simulink model "Espacio_Estados_sin_ROS_Comparacion"  (R2023a)
settings: Solver=VariableStepAuto  StartTime=0.0  StopTime=50  RelTol=1e-3
undefined symbols (not defined in the file): A, B, C, D, Ke, Ki
settings Model: Creator=mluser  LastModifiedBy=camarin
settings SolverCC: AlgebraicLoopSolver=TrustRegion
settings DataIOCC: ReturnWorkspaceOutputs=off
settings DebuggingCC: UnconnectedInputMsg=warning  UnconnectedOutputMsg=warning  UnconnectedLineMsg=warning
settings ModelReferenceCC: EnableRefExpFcnMdlSchedulingChecks=on
settings RTWCC: DLArmComputeVersion=19.05

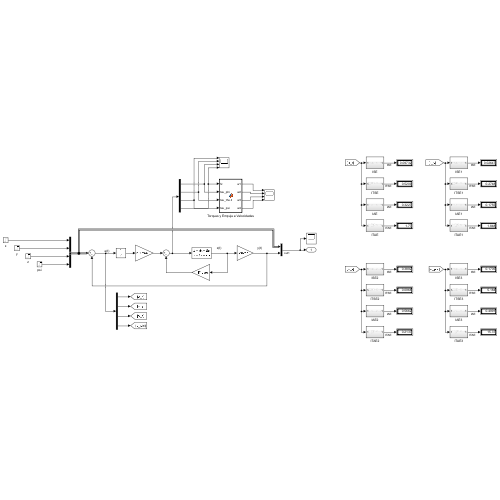
[thumbnail: Simulink's stored preview of the top-level diagram]
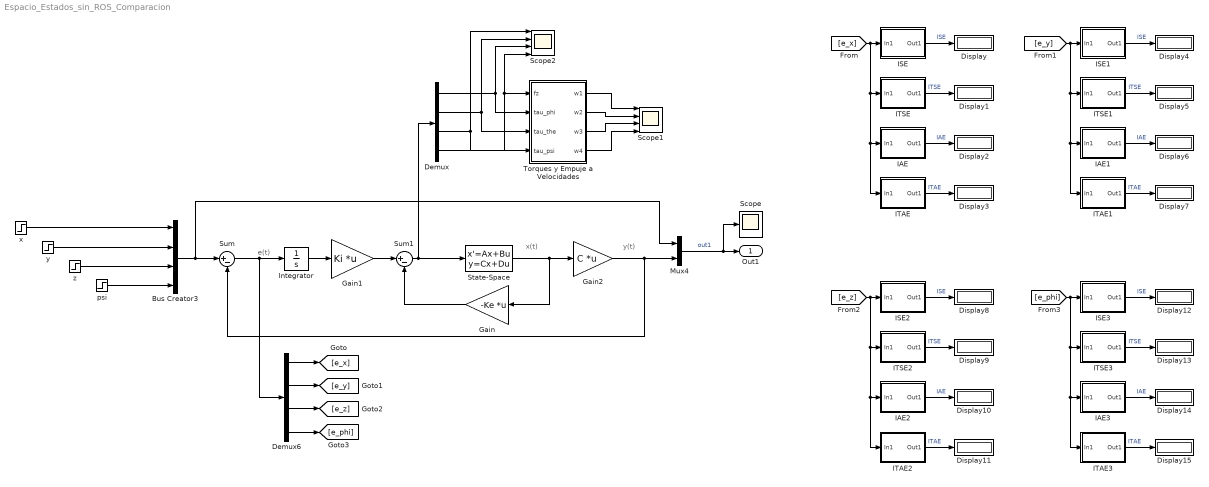
== system Espacio_Estados_sin_ROS_Comparacion ==
  note: e(t)
  note: y(t)
  note: x(t)
  Bus Creator3 : BusCreator  Inputs=4
  Demux : Demux
  Demux6 : Demux
  Display{,1..15} (16 alike) : Display
  Gain : Gain  Gain=-Ke  Multiplication=Matrix(K*u) (u vector)
  Gain1 : Gain  Gain=Ki  Multiplication=Matrix(K*u) (u vector)
  Gain2 : Gain  Gain=C  Multiplication=Matrix(K*u) (u vector)
  IAE : Subsystem
  IAE1 : Subsystem
  IAE2 : Subsystem
  IAE3 : Subsystem
  ISE : Subsystem
  ISE1 : Subsystem
  ISE2 : Subsystem
  ISE3 : Subsystem
  ITAE : Subsystem
  ITAE1 : Subsystem
  ITAE2 : Subsystem
  ITAE3 : Subsystem
  ITSE : Subsystem
  ITSE1 : Subsystem
  ITSE2 : Subsystem
  ITSE3 : Subsystem
  Integrator : Integrator
  Mux4 : Mux  Inputs=2
  Scope : Scope
  Scope1 : Scope  NumInputPorts=4
  Scope2 : Scope  NumInputPorts=4
  State-Space : StateSpace  A=A  B=B  C=eye(12)  D=D  InitialCondition=0  ParameterTunability=Unconstrained
  Sum : Sum  Inputs=|+-
  Sum1 : Sum  Inputs=|+-
  Torques y Empuje a Velocidades : MATLAB Function  TreatAsAtomicUnit=on
  psi : Step  Time=30  After=30*pi/180  SampleTime=0
  x : Step  Time=5  After=0.4  SampleTime=0
  y : Step  Time=10  After=0.2  SampleTime=0
  z : Step  Time=0  SampleTime=0
  Out1 : Outport
  wires:
  State-Space/1 -> Gain2/1, Gain/1
  Mux4/1 -> Scope/1, Out1/1  "out1"
  x/1 -> Bus Creator3/1
  z/1 -> Bus Creator3/3
  Bus Creator3/1 -> Sum/1, Mux4/1
  y/1 -> Bus Creator3/2
  psi/1 -> Bus Creator3/4
  Sum/1 -> Demux6/1, Integrator/1
  Sum1/1 -> Demux/1, State-Space/1
  Gain2/1 -> Sum/2, Mux4/2
  Gain/1 -> Sum1/2
  Integrator/1 -> Gain1/1
  Gain1/1 -> Sum1/1
  Torques y Empuje a Velocidades/1(w1) -> Scope1/1
  Torques y Empuje a Velocidades/2(w2) -> Scope1/2
  Torques y Empuje a Velocidades/3(w3) -> Scope1/3
  Torques y Empuje a Velocidades/4(w4) -> Scope1/4
  Demux/1 -> Scope2/3, Torques y Empuje a Velocidades/2(tau_phi)
  Demux/2 -> Scope2/2, Torques y Empuje a Velocidades/3(tau_the)
  Demux/3 -> Scope2/1, Torques y Empuje a Velocidades/4(tau_psi)
  Demux/4 -> Scope2/4, Torques y Empuje a Velocidades/1(fz)
  ISE1/1(Out1) -> Display4/1  "ISE"
  IAE1/1(Out1) -> Display6/1  "IAE"
  [e_z] -> ITAE2/1(In1), IAE2/1(In1), ITSE2/1(In1), ISE2/1(In1)
  ISE2/1(Out1) -> Display8/1  "ISE"
  ITSE2/1(Out1) -> Display9/1  "ITSE"
  ITSE3/1(Out1) -> Display13/1  "ITSE"
  [e_phi] -> ITAE3/1(In1), IAE3/1(In1), ITSE3/1(In1), ISE3/1(In1)
  ITAE2/1(Out1) -> Display11/1  "ITAE"
  IAE3/1(Out1) -> Display14/1  "IAE"
  IAE2/1(Out1) -> Display10/1  "IAE"
  IAE/1(Out1) -> Display2/1  "IAE"
  ITAE/1(Out1) -> Display3/1  "ITAE"
  [e_y] -> ITAE1/1(In1), IAE1/1(In1), ITSE1/1(In1), ISE1/1(In1)
  ITSE/1(Out1) -> Display1/1  "ITSE"
  ISE3/1(Out1) -> Display12/1  "ISE"
  ISE/1(Out1) -> Display/1  "ISE"
  ITAE3/1(Out1) -> Display15/1  "ITAE"
  ITSE1/1(Out1) -> Display5/1  "ITSE"
  ITAE1/1(Out1) -> Display7/1  "ITAE"
  [e_x] -> ITAE/1(In1), IAE/1(In1), ITSE/1(In1), ISE/1(In1)
  Demux6/1 -> [e_x]
  Demux6/2 -> [e_y]
  Demux6/3 -> [e_z]
  Demux6/4 -> [e_phi]

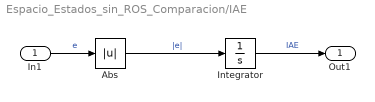
== system Espacio_Estados_sin_ROS_Comparacion/IAE ==
  In1 : Inport
  Abs : Abs  SaturateOnIntegerOverflow=off
  Integrator : Integrator
  Out1 : Outport
  wires:
  Integrator/1 -> Out1/1  "IAE"
  In1/1 -> Abs/1  "e"
  Abs/1 -> Integrator/1  "|e|"

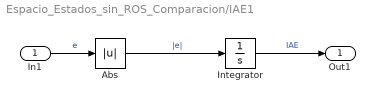
== system Espacio_Estados_sin_ROS_Comparacion/IAE1 ==
  In1 : Inport
  Abs : Abs  SaturateOnIntegerOverflow=off
  Integrator : Integrator
  Out1 : Outport
  wires:
  Integrator/1 -> Out1/1  "IAE"
  In1/1 -> Abs/1  "e"
  Abs/1 -> Integrator/1  "|e|"

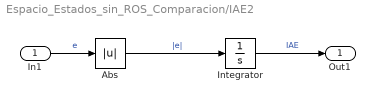
== system Espacio_Estados_sin_ROS_Comparacion/IAE2 ==
  In1 : Inport
  Abs : Abs  SaturateOnIntegerOverflow=off
  Integrator : Integrator
  Out1 : Outport
  wires:
  Integrator/1 -> Out1/1  "IAE"
  In1/1 -> Abs/1  "e"
  Abs/1 -> Integrator/1  "|e|"

== system Espacio_Estados_sin_ROS_Comparacion/IAE3 ==
  In1 : Inport
  Abs : Abs  SaturateOnIntegerOverflow=off
  Integrator : Integrator
  Out1 : Outport
  wires:
  Integrator/1 -> Out1/1  "IAE"
  In1/1 -> Abs/1  "e"
  Abs/1 -> Integrator/1  "|e|"

== system Espacio_Estados_sin_ROS_Comparacion/ISE ==
  In1 : Inport
  Integrator : Integrator
  Product : Product
  Out1 : Outport
  wires:
  In1/1 -> Product/2, Product/1  "e"
  Product/1 -> Integrator/1  "e^2"
  Integrator/1 -> Out1/1  "ISE"

== system Espacio_Estados_sin_ROS_Comparacion/ISE1 ==
  In1 : Inport
  Integrator : Integrator
  Product : Product
  Out1 : Outport
  wires:
  In1/1 -> Product/2, Product/1  "e"
  Product/1 -> Integrator/1  "e^2"
  Integrator/1 -> Out1/1  "ISE"

== system Espacio_Estados_sin_ROS_Comparacion/ISE2 ==
  In1 : Inport
  Integrator : Integrator
  Product : Product
  Out1 : Outport
  wires:
  In1/1 -> Product/2, Product/1  "e"
  Product/1 -> Integrator/1  "e^2"
  Integrator/1 -> Out1/1  "ISE"

== system Espacio_Estados_sin_ROS_Comparacion/ISE3 ==
  In1 : Inport
  Integrator : Integrator
  Product : Product
  Out1 : Outport
  wires:
  In1/1 -> Product/2, Product/1  "e"
  Product/1 -> Integrator/1  "e^2"
  Integrator/1 -> Out1/1  "ISE"

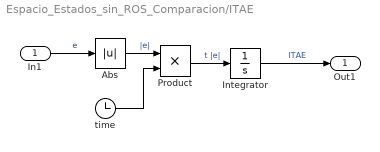
== system Espacio_Estados_sin_ROS_Comparacion/ITAE ==
  In1 : Inport
  Abs : Abs  SaturateOnIntegerOverflow=off
  Integrator : Integrator
  Product : Product
  time : Clock
  Out1 : Outport
  wires:
  In1/1 -> Abs/1  "e"
  Integrator/1 -> Out1/1  "ITAE"
  time/1 -> Product/2
  Abs/1 -> Product/1  "|e|"
  Product/1 -> Integrator/1  "t |e|"

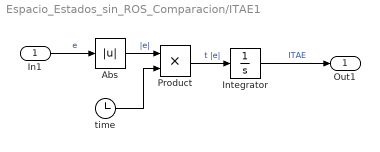
== system Espacio_Estados_sin_ROS_Comparacion/ITAE1 ==
  In1 : Inport
  Abs : Abs  SaturateOnIntegerOverflow=off
  Integrator : Integrator
  Product : Product
  time : Clock
  Out1 : Outport
  wires:
  In1/1 -> Abs/1  "e"
  Integrator/1 -> Out1/1  "ITAE"
  time/1 -> Product/2
  Abs/1 -> Product/1  "|e|"
  Product/1 -> Integrator/1  "t |e|"

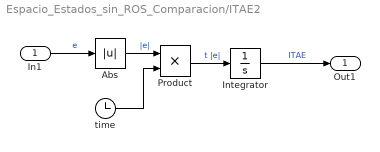
== system Espacio_Estados_sin_ROS_Comparacion/ITAE2 ==
  In1 : Inport
  Abs : Abs  SaturateOnIntegerOverflow=off
  Integrator : Integrator
  Product : Product
  time : Clock
  Out1 : Outport
  wires:
  In1/1 -> Abs/1  "e"
  Integrator/1 -> Out1/1  "ITAE"
  time/1 -> Product/2
  Abs/1 -> Product/1  "|e|"
  Product/1 -> Integrator/1  "t |e|"

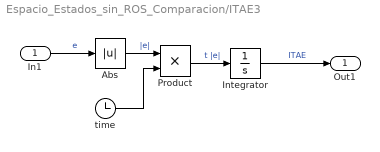
== system Espacio_Estados_sin_ROS_Comparacion/ITAE3 ==
  In1 : Inport
  Abs : Abs  SaturateOnIntegerOverflow=off
  Integrator : Integrator
  Product : Product
  time : Clock
  Out1 : Outport
  wires:
  In1/1 -> Abs/1  "e"
  Integrator/1 -> Out1/1  "ITAE"
  time/1 -> Product/2
  Abs/1 -> Product/1  "|e|"
  Product/1 -> Integrator/1  "t |e|"

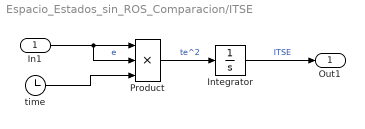
== system Espacio_Estados_sin_ROS_Comparacion/ITSE ==
  In1 : Inport
  Integrator : Integrator
  Product : Product  Inputs=3
  time : Clock
  Out1 : Outport
  wires:
  Integrator/1 -> Out1/1  "ITSE"
  In1/1 -> Product/1, Product/2  "e"
  time/1 -> Product/3
  Product/1 -> Integrator/1  "te^2"

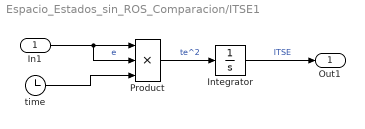
== system Espacio_Estados_sin_ROS_Comparacion/ITSE1 ==
  In1 : Inport
  Integrator : Integrator
  Product : Product  Inputs=3
  time : Clock
  Out1 : Outport
  wires:
  Integrator/1 -> Out1/1  "ITSE"
  In1/1 -> Product/1, Product/2  "e"
  time/1 -> Product/3
  Product/1 -> Integrator/1  "te^2"

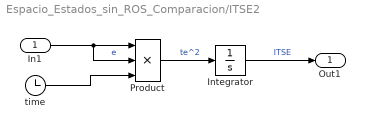
== system Espacio_Estados_sin_ROS_Comparacion/ITSE2 ==
  In1 : Inport
  Integrator : Integrator
  Product : Product  Inputs=3
  time : Clock
  Out1 : Outport
  wires:
  Integrator/1 -> Out1/1  "ITSE"
  In1/1 -> Product/1, Product/2  "e"
  time/1 -> Product/3
  Product/1 -> Integrator/1  "te^2"

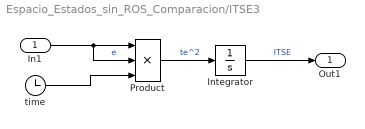
== system Espacio_Estados_sin_ROS_Comparacion/ITSE3 ==
  In1 : Inport
  Integrator : Integrator
  Product : Product  Inputs=3
  time : Clock
  Out1 : Outport
  wires:
  Integrator/1 -> Out1/1  "ITSE"
  In1/1 -> Product/1, Product/2  "e"
  time/1 -> Product/3
  Product/1 -> Integrator/1  "te^2"

== matlab function Espacio_Estados_sin_ROS_Comparacion/Torques y Empuje a Velocidades ==
  data: fz input; w1 output; tau_phi input; w2 output; w3 output; w4 output; tau_the input; tau_psi input
function [w1,w2,w3,w4] = H(fz,tau_phi,tau_the,tau_psi)
%         Salidas          Entradas

% Constantes 
l = 0.2;    % m
kf = 0.007; % Nm/A
km = 0.8;   % V/kRPM

% Matriz H
H = [kf     kf      kf      kf;
     0      l*kf    0       -l*kf;
     -l*kf  0       l*kf    0;  
     km     -km     km      -km];
 
% Inversa de H
H_inversa = inv(H);

% Vector de entrada
Torques = [fz;
           tau_phi;
           tau_the;
           tau_psi];
       
% Vector de salida      
Wi2 = H_inversa * Torques;


% Velocidades angulares al cuadrado
w1 = sqrt(abs(Wi2(1))) + 25;
w2 = sqrt(abs(Wi2(2))) + 25;
w3 = sqrt(abs(Wi2(3))) + 25;
w4 = sqrt(abs(Wi2(4))) + 25;


% Saturación de las velocidades angulares
RPM = 1020;
wmax = RPM*2*pi/60;
if w1>wmax
    w1 = wmax;
end
if w2>wmax
    w2 = wmax;
end
if w3>wmax
    w3 = wmax;
end
if w4>wmax
    w4 = wmax;
end
